simulink model "controlled"  (Simulink 7.9)
settings: Solver=ode45  StartTime=0.0  StopTime=2000  RelTol=1e-3
settings Model: Creator=kr2112  LastModifiedBy=kr2112
settings DebuggingCC: MaxConsecutiveZCsMsg=none

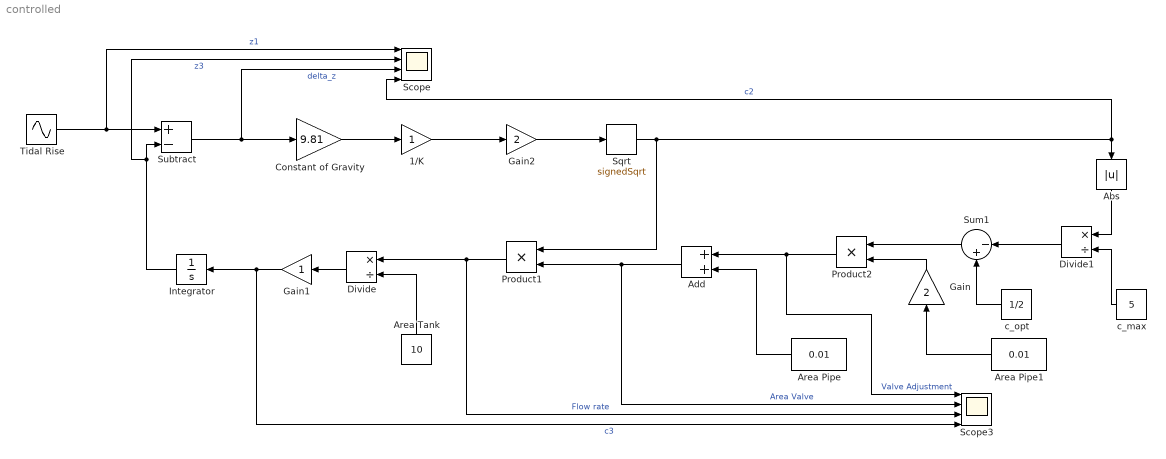
== system controlled ==
  1/K : Gain
  Abs : Abs
  Add : Sum
  Area Pipe : Constant  Value=0.01
  Area Pipe1 : Constant  Value=0.01
  Area Tank : Constant  Value=10
  Constant of Gravity : Gain  Gain=9.81
  Divide : Product  Inputs=*/
  Divide1 : Product  Inputs=*/
  Gain : Gain  Gain=2
  Gain1 : Gain
  Gain2 : Gain  Gain=2
  Integrator : Integrator
  Product1 : Product  RndMeth=Zero
  Product2 : Product  RndMeth=Zero
  Scope : Scope  NumInputPorts=4
      settings: YMin=0~-0.00025~0~0  YMax=1~0.0025~1~4.5
  Scope3 : Scope  NumInputPorts=4
      settings: YMin=-5~-5~-5~-5  YMax=5~5~5~5  SaveName=ScopeData3
  Sqrt : Sqrt  Operator=signedSqrt  SaturateOnIntegerOverflow=on
  Subtract : Sum  Inputs=+-
  Sum1 : Sum  Inputs=|-+
  Tidal Rise : Sin  Frequency=0.0083  SampleTime=0
  c_max : Constant  Value=5
  c_opt : Constant  Value=1/2
  wires:
  Constant of Gravity/1 -> 1/K/1
  1/K/1 -> Gain2/1
  Sqrt/1 -> Product1/1, Scope/4, Abs/1  "c2"
  Subtract/1 -> Constant of Gravity/1, Scope/3  "delta_z"
  Tidal Rise/1 -> Subtract/1, Scope/1  "z1"
  Gain2/1 -> Sqrt/1
  Product1/1 -> Divide/1, Scope3/3  "Flow rate"
  Area Tank/1 -> Divide/2
  c_opt/1 -> Sum1/2
  Add/1 -> Product1/2, Scope3/2  "Area Valve"
  Area Pipe/1 -> Add/2
  Divide/1 -> Gain1/1
  Gain1/1 -> Scope3/4, Integrator/1  "c3"
  Sum1/1 -> Product2/1
  Abs/1 -> Divide1/1
  Divide1/1 -> Sum1/1
  c_max/1 -> Divide1/2
  Area Pipe1/1 -> Gain/1
  Gain/1 -> Product2/2
  Product2/1 -> Add/1, Scope3/1  "Valve Adjustment"
  Integrator/1 -> Subtract/2, Scope/2  "z3"
